simulink model "DVM_Nikola_final"  (Simulink 7.6)
settings: Solver=ode45  StartTime=0.0  StopTime=5  RelTol=1e-3
libraries: simulink x1
settings Model: Creator=nnoxon  LastModifiedBy=Nikola
settings DebuggingCC: SolverPrmCheckMsg=none

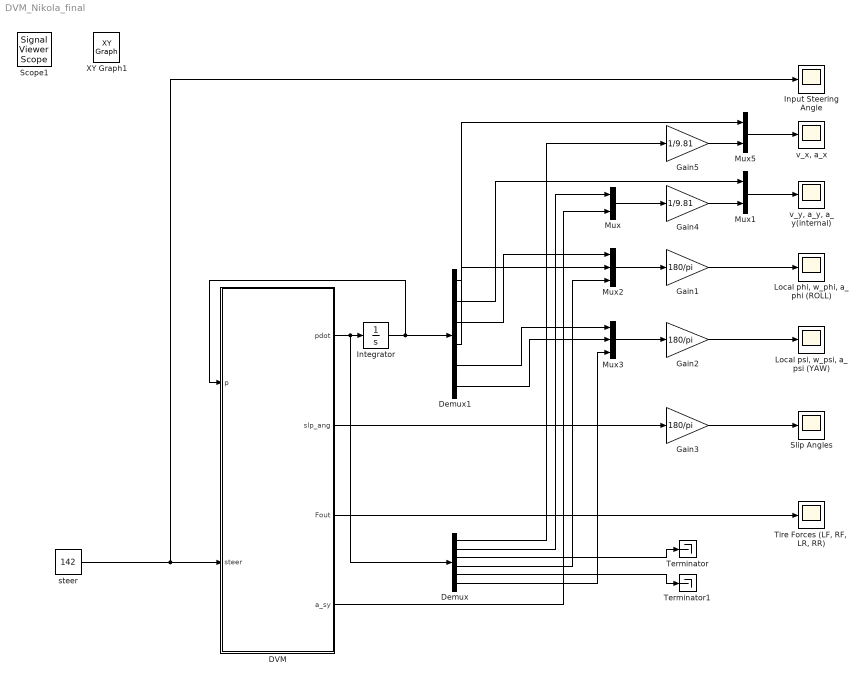
== system DVM_Nikola_final ==
  DVM : Stateflow chart  TreatAsAtomicUnit=on
  Demux : Demux  Outputs=6
  Demux1 : Demux  Outputs=6
  Gain1 : Gain  Gain=180/pi
  Gain2 : Gain  Gain=180/pi
  Gain3 : Gain  Gain=180/pi
  Gain4 : Gain  Gain=1/9.81
  Gain5 : Gain  Gain=1/9.81
  Input Steering Angle : Scope
      settings: SaveName=ScopeData7
  Integrator : Integrator  InitialCondition=[11.11,0,0,0,0,0]
  "Local phi, w_phi, a_phi (ROLL)" : Scope
      settings: TimeRange=4.975412376233293  YMin=-15  SaveName=ScopeData2
  "Local psi, w_psi, a_psi (YAW)" : Scope
      settings: TimeRange=4.986678507992896  YMin=-3.993902439024392  YMax=40.21341463414633  SaveName=ScopeData3
  Mux : Mux  Inputs=2
  Mux1 : Mux  Inputs=2
  Mux2 : Mux  Inputs=3
  Mux3 : Mux  Inputs=3
  Mux5 : Mux  Inputs=2
  Slip Angles : Scope
  Terminator : Terminator
  Terminator1 : Terminator
  "Tire Forces (LF, RF, LR, RR)" : Scope
      settings: SaveName=ScopeData6
  steer : Constant  Value=142
  "v_x, a_x" : Scope
      settings: YMin=-5e-005  YMax=0.001  SaveName=ScopeData5
  "v_y, a_y, a_y(internal)" : Scope
      settings: TimeRange=5  YMin=-100000  YMax=110000
  Scope1 : SignalViewerScope  IOType=viewer  RefreshTime=0.035000
  XY Graph1 : simulink/Sinks/XY Graph  IOType=viewer  SystemSampleTime=-1  xmin=-1  xmax=1  ymin=-1  ymax=1  st=-1
  wires:
  DVM/2(slp_ang) -> Gain3/1
  Gain3/1 -> Slip Angles/1
  Mux3/1 -> Gain2/1
  Mux2/1 -> Gain1/1
  Mux/1 -> Gain4/1
  Gain4/1 -> Mux1/2
  Mux1/1 -> "v_y, a_y, a_y(internal)"/1
  Gain1/1 -> "Local phi, w_phi, a_phi (ROLL)"/1
  Gain2/1 -> "Local psi, w_psi, a_psi (YAW)"/1
  Demux1/6 -> Mux3/2
  Demux1/5 -> Mux3/1
  Gain5/1 -> Mux5/2
  Mux5/1 -> "v_x, a_x"/1
  Demux/1 -> Gain5/1
  Demux/4 -> Mux2/3
  Demux/2 -> Mux/1
  Demux1/2 -> Mux1/1
  Demux1/1 -> Mux5/1
  Demux1/4 -> Mux2/2
  Demux1/3 -> Mux2/1
  DVM/1(pdot) -> Integrator/1, Demux/1
  Integrator/1 -> DVM/1(p), Demux1/1
  DVM/3(Fout) -> "Tire Forces (LF, RF, LR, RR)"/1
  steer/1 -> DVM/2(steer), Input Steering Angle/1
  Demux/6 -> Mux3/3
  DVM/4(a_sy) -> Mux/2
  Demux/3 -> Terminator/1
  Demux/5 -> Terminator1/1

== matlab function DVM ==
  data: p input double; pdot output double; steer input double; slp_ang output double; Fout output double; a_sy output double
function [pdot,slp_ang,Fout,a_sy] = DVM(p,steer)
 
%---------------------------------------%
%CONSTANTS
%---------------------------------------%
g = 9.81;
%---------------------------------------%


%---------------------------------------%
%CURRENT STATE/INPUT
%---------------------------------------%
v_x = p(1);
v_y = p(2);
phi = p(3);
phi_d = p(4);
psi = p(5);
psi_d = p(6);

d_steer = steer;
%---------------------------------------%


%---------------------------------------%
%VEHICLE PAREMETERS
%---------------------------------------%
%lengths
l_fs = 1.01476;             %length from sprung mass CG to front suspension
l_rs = 1.67524;             %length from sprung mass CG to rear suspension
t_f = 1.540;                %front vehicle width
t_r = 1.530;                %rear vehicle width
h_f = 0.130;                %height from ground to front suspension
h_r = 0.110;                %height from ground to rear suspension
h_cgs = 0.567851;           %height from ground to sprung CG
h_cguf = 0.320;             %height from ground to front unsprung CG
h_cgur = 0.320;             %height from ground to rear unsprung CG

%mass/inertia
M = 1704.7;                 %total vehicle mass
M_uf = 98.1;                %unsprung front mass
M_ur = 79.7;                %unsprung rear mass
I_xxs = 440.911;            %sprung XX inertia
I_xys = 0;                  %sprung XY inertia
I_xzs = 7.54097;            %sprung XZ inertia
I_yys = 2498.900;           %sprung YY inertia
I_yzs = 0;                  %sprung yz inertia
I_zzs = 2619.28;            %sprung ZZ inertia
I_zzuf = M_uf*(t_f/2)^2;    %front unsprung ZZ inertia
I_zzur = M_ur*(t_r/2)^2;    %rear unsprung ZZ inertia
I_tlf = 0.99;               %front left tire inertia
I_trf = 0.99;               %front right tire inertia
I_tlr = 0.99;               %rear left tire inertia
I_trr = 0.99;               %rear right tire inertia

%tire slip curve coordinates (slip-%, mu)
vary =  [0.0 0.0
        0.08 0.4
        0.15 0.6
         0.3 0.8
         1.0 0.4];

%spring/dampers
K_spf = 27.85; %N/mm
K_spr = 18.16; %N/mm
 
B_f = 2.9915; %N-s/mm
B_r = 2.9915; %N-s/mm
 
%anti_roll bars
K_rf = 384.0*180/pi; %Nm/rad
K_rr = 344.4*180/pi;

%steering-to-wheel angle ratio
K_sr = 15.97;

%sprung mass
M_s = M - M_uf - M_ur;

%calculated dimensions
L = l_fs + l_rs;                    %distance from front to rear suspension
l_cgs = (M_ur*l_rs - M_uf*l_fs)/M;  %distance from vehicle CG to sprung CG
l_f = l_fs + l_cgs;                 %distance from vehicle CG to front suspension
l_r = l_rs - l_cgs;                 %distance from vehicle CG to rear suspension
h_o = h_f + l_f*(h_r - h_f)/L;      %height from ground to roll axis
h_s = h_cgs - h_o;                  %height from roll axis to sprung CG
h_uf = h_cguf - h_o;                %height from roll axis to front suspension
h_ur = h_cgur - h_o;                %height from roll axis to rear suspension

%Tire Normal Forces
Fzlf = M*g*l_r/(2*L);               
Fzrf = M*g*l_r/(2*L);
Fzlr = M*g*l_f/(2*L);
Fzrr = M*g*l_f/(2*L);

%roll stiffness
K_phif = 0.766*K_spf*1000*t_f^2/2 + K_rf;%
K_phir = 0.827*K_spr*1000*t_r^2/2 + K_rr;%
 
%roll damping
B_phif = 0.766*B_f*1000*t_f^2/2; %Nm-s/rad
B_phir = 0.827*B_r*1000*t_r^2/2;
%---------------------------------------%

%---------------------------------------%
%ROTATION MATRIX
%---------------------------------------%
ROT = [1            0           0;
       0     cos(phi)    sin(phi);
       0    -sin(phi)   cos(phi)];
 
I_b = [    I_xxs+M_s*h_s^2                      I_xys   I_xzs+M_s*h_s*l_cgs
                     I_xys  I_yys+M_s*(h_s^2+l_cgs^2)                 I_yzs
       I_xzs+M_s*h_s*l_cgs                      I_yzs   I_zzs+M_s*l_cgs^2];
   
I_c = ROT*I_b*ROT'; %chassis M.o.I. tensor
 
I_zzus = M_uf*l_f^2 + ...
         M_ur*l_r^2 + ...
         I_zzuf + I_zzur;
 
I_zzo = I_c(3,3) + I_zzus; %effective I_zz
%---------------------------------------%

% %---------------------------------------%
% %DYNAMIC WEIGHT TRANSFER FORCES
% %---------------------------------------%
% %internal accelerations
% a_sx = a_x - psi_d*v_y ...
%      - 2*h_s*phi_d*psi_d*cos(phi) ...
%      - l_cgs*psi_d^2;
% a_sy = a_y + psi_d*v_x ...
%      + l_cgs*psi_dd ...
%      + h_s*cos(phi)*phi_dd ...
%      - h_s*phi_d^2*sin(phi) ...
%      - h_s*psi_d^2*sin(phi);
% a_ufx = a_x - l_f*psi_d^2;
% a_ufy = a_y + l_f*psi_dd;
% a_urx = a_x + l_r*psi_d^2;
% a_ury = a_y - l_r*psi_dd;
% 
% 
% Fzax = (M_s*h_s*a_sx + M_uf*h_uf*a_ufx + M_ur*h_ur*a_urx)/(2*L);
% 
% Fzayf = 1/t_f*(M_s*l_r*h_f/L*a_sy + M_uf*h_uf*a_ufy);
% Fzayr = 1/t_r*(M_s*l_f*h_r/L*a_sy + M_ur*h_ur*a_ury);
% 
% Fzphif = -1/t_f*(K_phif*phi + B_phif*phi_d);
% Fzphir = -1/t_r*(K_phir*phi + B_phir*phi_d);
%
% Fzlf = M*g*l_r/(2*L) - Fzax - Fzayf + Fzphif;
% Fzrf = M*g*l_r/(2*L) - Fzax + Fzayf - Fzphif;
% Fzlr = M*g*l_f/(2*L) + Fzax - Fzayr + Fzphir;
% Fzrr = M*g*l_f/(2*L) + Fzax + Fzayr - Fzphir;
% %---------------------------------------%
 
%---------------------------------------%
%TIRE LONGITUDINAL/CORNERING SPEEDS
%---------------------------------------%
%left front wheel velocity
vx_lf = v_x + psi_d*t_f/2;
vy_lf = v_y + psi_d*l_f;
 
%right front wheel velocity
vx_rf = v_x - psi_d*t_f/2;
vy_rf = v_y + psi_d*l_f;
 
%left rear wheel velocity
vx_lr = v_x + psi_d*t_r/2;
vy_lr = v_y - psi_d*l_r;
 
%right rear wheel velocity
vx_rr = v_x - psi_d*t_r/2;
vy_rr = v_y - psi_d*l_r;  
%---------------------------------------%

%---------------------------------------%
%SLIP ANGLES
%---------------------------------------%
%steer angle in radians
delta = d_steer/(180*K_sr)*pi;

% Tire longitudinal and cornering velocities
vc_lf = vy_lf*cos(delta) - vx_lf*sin(delta);
vl_lf = vy_lf*sin(delta) + vx_lf*cos(delta);

vc_rf = vy_rf*cos(delta) - vx_rf*sin(delta);
vl_rf = vy_rf*sin(delta) + vx_rf*cos(delta);

vc_lr = vy_lr;
vl_lr = vx_lr;

vc_rr = vy_rr;
vl_rr = vx_rr;

% Slip angles
a_lf = atan(vc_lf/vl_lf);
a_rf = atan(vc_rf/vl_rf);
a_lr = atan(vc_lr/vl_lr);
a_rr = atan(vc_rr/vl_rr);

slp_ang = [a_lf,a_rf,a_lr,a_rr];
%---------------------------------------%

%---------------------------------------%
%TIRE LONGITUDINAL/CORNERING FORCES
%---------------------------------------%
C_alf = vary(2,2)/vary(2,1)*Fzlf;
C_arf = vary(2,2)/vary(2,1)*Fzrf;
C_alr = vary(2,2)/vary(2,1)*Fzlr;
C_arr = vary(2,2)/vary(2,1)*Fzrr;

Fxtlf = 0;
Fxtrf = 0;
Fxtlr = 0;
Fxtrr = 0;
 
Fytlf = -a_lf*C_alf;
Fytrf = -a_rf*C_arf;
Fytlr = -a_lr*C_alr;
Fytrr = -a_rr*C_arr;
 
Fxlf = Fxtlf*cos(delta) - Fytlf*sin(delta);
Fxrf = Fxtrf*cos(delta) - Fytrf*sin(delta);
Fxlr = Fxtlr;
Fxrr = Fxtrr;
 
Fylf = Fytlf*cos(delta) + Fxtlf*sin(delta);
Fyrf = Fytrf*cos(delta) + Fxtrf*sin(delta);
Fylr = Fytlr;
Fyrr = Fytrr;
 
Fout = [Fylf,Fyrf,Fylr,Fyrr];
%---------------------------------------%

%---------------------------------------%
%TIRE TORQUES
%---------------------------------------%
T_phif = -K_phif*phi - B_phif*phi_d;
T_phir = -K_phir*phi - B_phir*phi_d;
%---------------------------------------%
 
%---------------------------------------%
%SUMMATION OF FORCES AND MOMENTS
%---------------------------------------%
sigFx   = Fxlf + Fxrf + Fxlr + Fxrr;
sigFy   = Fylf + Fyrf + Fylr + Fyrr;
sigTxs  = T_phif + T_phir - ...
          M_s*g*h_s*sin(phi);
sigTz   = (Fylf + Fyrf)*l_f - (Fylr + Fyrr)*l_r + ...
          t_f/2*(Fxlf - Fxrf) + t_r/2*(Fxlr - Fxrr);
%---------------------------------------%

%---------------------------------------%
%EQUATIONS OF MOTION
%---------------------------------------%
%mass matrix for coupled equations of motion
M11 = M;
M14  = M_s*h_s*sin(phi);
M22 = M;
M23 = -M_s*h_s*cos(phi);
M32 = M_s*h_s*cos(phi);
M33 = I_xxs+M_s*h_s^2*(1+cos(phi)^2);
M34 = (I_xzs+2*M_s*h_s*l_cgs)*cos(phi);
M41 = M_s*h_s*sin(phi);
M43 = (I_xzs+M_s*h_s*l_cgs)*cos(phi);
M44 = I_zzo;

Mass_Matrix =   [M11     0     0   M14
                   0   M22   M23     0
                   0   M32   M33   M34
                 M41     0   M43   M44];

%coupled equations of motion
A1 = -2*M_s*h_s*cos(phi);
B1 = -M_s*h_s*sin(phi);
C1 = (I_xzs+M_s*h_s*l_cgs)*sin(phi);
C2 = (I_zzs - I_yys)*sin(phi)*cos(phi);
C3 = M_s*h_s^2*sin(phi)*cos(phi);
C4 = -M_s*h_s*cos(phi);
D1 = -(I_xzs+M_s*h_s*l_cgs)*sin(phi);
D2 = -(I_zzs - I_yys - M_s*h_s^2)*sin(phi)*cos(phi);

F_c = zeros(4,1);             

F_c(1) = sigFx  + A1*phi_d*psi_d;
F_c(2) = sigFy  + B1*(phi_d^2 + psi_d^2);
F_c(3) = sigTxs + C1*phi_d*psi_d + C2*psi_d^2 + C3*phi_d^2 + C4*psi_d*v_x;
F_c(4) = sigTz  + D1*phi_d^2     + D2*psi_d*phi_d;

%decouple the EoM
F_u = Mass_Matrix^-1*F_c; 

%extract the left hand side of the EoM
a_x = F_u(1);
a_y = F_u(2);
phi_dd = F_u(3);
psi_dd = F_u(4);
%---------------------------------------%

%---------------------------------------%
% STATE TRAJECTORY OUTPUT
%---------------------------------------%
pdot = [a_x;a_y;phi_d;phi_dd;psi_d;psi_dd];
%---------------------------------------%

a_sy = a_y + psi_d*v_x ...
     + l_cgs*psi_dd ...
     + h_s*cos(phi)*phi_dd ...
     - h_s*phi_d^2*sin(phi) ...
     - h_s*psi_d^2*sin(phi);
%end
